simulink model "controller"  (R2016b)
settings: Solver=VariableStepAuto  StartTime=0.0  StopTime=10.0  RelTol=1e-3
values from neighbouring files (symbols this model uses):
  MAX_TORQUE_OUTPUT = 500    [Control_Init.m]
  PID_D = 0.01    [Control_Init.m]
  PID_I = 0.0    (= 0)    [Control_Init.m]
  PID_P = 0.2    [Control_Init.m]
undefined symbols (not defined in the file or in its folder): PID_FN
libraries: simulink x2
settings Model: Creator=root  LastModifiedBy=root
settings DataIOCC: SignalLogging=off
settings HardwareCC: ProdBitPerLong=64  ProdHWDeviceType=Intel->x86-64 (Linux 64)
settings RTWCC: GenCodeOnly=on  PackageGeneratedCodeAndArtifacts=on  PackageName=library

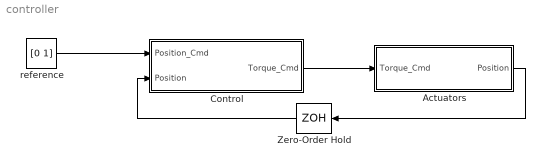
== system controller ==
  Actuators : Subsystem
  Control : Subsystem
  Zero-Order Hold : ZeroOrderHold  SampleTime=0.001
  reference : Constant  Value=[0 1]
  wires:
  Control/1(Torque_Cmd) -> Actuators/1(Torque_Cmd)
  Actuators/1(Position) -> Zero-Order Hold/1
  reference/1 -> Control/1(Position_Cmd)
  Zero-Order Hold/1 -> Control/2(Position)

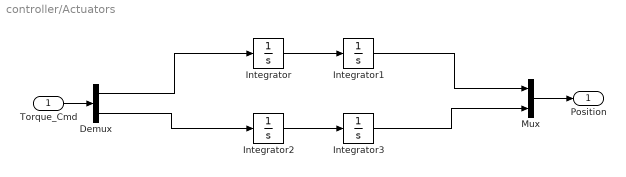
== system controller/Actuators ==
  Torque_Cmd : Inport
  Demux : Demux  Outputs=2
  Integrator : Integrator  ContinuousStateAttributes='velocity_1'
  Integrator1 : Integrator  ContinuousStateAttributes='position_1'
  Integrator2 : Integrator  ContinuousStateAttributes='velocity_2'
  Integrator3 : Integrator  ContinuousStateAttributes='position_2'
  Mux : Mux  Inputs=2
  Position : Outport
  wires:
  Integrator/1 -> Integrator1/1
  Integrator2/1 -> Integrator3/1
  Demux/1 -> Integrator/1
  Mux/1 -> Position/1
  Integrator1/1 -> Mux/1
  Integrator3/1 -> Mux/2
  Demux/2 -> Integrator2/1
  Torque_Cmd/1 -> Demux/1

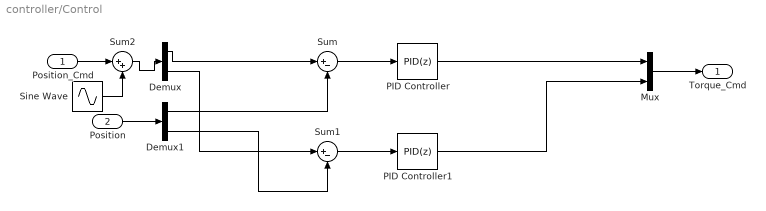
== system controller/Control ==
  Position_Cmd : Inport  PortDimensions=n_actuators
  Position : Inport  Port=2  PortDimensions=n_actuators
  Demux : Demux  Outputs=n_actuators
  Demux1 : Demux  Outputs=n_actuators
  Mux : Mux  Inputs=n_actuators
  PID Controller : simulink/Continuous/PID Controller  Controller=PID  TimeDomain=Discrete-time  SampleTime=-1  IntegratorMethod=Forward Euler  FilterMethod=Forward Euler  Form=Parallel  UseFilter=on  ControllerParametersSource=internal  P=PID_P  I=PID_I  D=PID_D  N=PID_FN  InitialConditionSource=internal  InitialConditionForIntegrator=0  InitialConditionForFilter=0  ExternalReset=none  LimitOutput=on  UpperSaturationLimit=MAX_TORQUE_OUTPUT  LowerSaturationLimit=-MAX_TORQUE_OUTPUT  LinearizeAsGain=on  AntiWindupMode=clamping  Kb=1  TrackingMode=off  Kt=1  PParamMin=[]  PParamMax=[]  IParamMin=[]  IParamMax=[]  DParamMin=[]  DParamMax=[]  NParamMin=[]  NParamMax=[]  KbParamMin=[]  KbParamMax=[]  KtParamMin=[]  KtParamMax=[]  POutMin=[]  POutMax=[]  IOutMin=[]  IOutMax=[]  DOutMin=[]  DOutMax=[]  NOutMin=[]  NOutMax=[]  KbOutMin=[]  KbOutMax=[]  KtOutMin=[]  KtOutMax=[]  IntegratorOutMin=[]  IntegratorOutMax=[]  FilterOutMin=[]  FilterOutMax=[]  SumOutMin=[]  SumOutMax=[]  SumI1OutMin=[]  SumI1OutMax=[]  SumI2OutMin=[]  SumI2OutMax=[]  SumI3OutMin=[]  SumI3OutMax=[]  SumDOutMin=[]  SumDOutMax=[]  SaturationOutMin=[]  SaturationOutMax=[]  IntegratorContinuousStateAttributes=''  IntegratorStateMustResolveToSignalObject=off  IntegratorRTWStateStorageClass=Auto  FilterContinuousStateAttributes=''  FilterStateMustResolveToSignalObject=off  FilterRTWStateStorageClass=Auto  DifferentiatorICPrevScaledInput=0  DifferentiatorOutMin=[]  DifferentiatorOutMax=[]
  PID Controller1 : simulink/Continuous/PID Controller  Controller=PID  TimeDomain=Discrete-time  SampleTime=-1  IntegratorMethod=Forward Euler  FilterMethod=Forward Euler  Form=Parallel  UseFilter=on  ControllerParametersSource=internal  P=PID_P  I=PID_I  D=PID_D  N=PID_FN  InitialConditionSource=internal  InitialConditionForIntegrator=0  InitialConditionForFilter=0  ExternalReset=none  LimitOutput=on  UpperSaturationLimit=MAX_TORQUE_OUTPUT  LowerSaturationLimit=-MAX_TORQUE_OUTPUT  LinearizeAsGain=on  AntiWindupMode=clamping  Kb=1  TrackingMode=off  Kt=1  PParamMin=[]  PParamMax=[]  IParamMin=[]  IParamMax=[]  DParamMin=[]  DParamMax=[]  NParamMin=[]  NParamMax=[]  KbParamMin=[]  KbParamMax=[]  KtParamMin=[]  KtParamMax=[]  POutMin=[]  POutMax=[]  IOutMin=[]  IOutMax=[]  DOutMin=[]  DOutMax=[]  NOutMin=[]  NOutMax=[]  KbOutMin=[]  KbOutMax=[]  KtOutMin=[]  KtOutMax=[]  IntegratorOutMin=[]  IntegratorOutMax=[]  FilterOutMin=[]  FilterOutMax=[]  SumOutMin=[]  SumOutMax=[]  SumI1OutMin=[]  SumI1OutMax=[]  SumI2OutMin=[]  SumI2OutMax=[]  SumI3OutMin=[]  SumI3OutMax=[]  SumDOutMin=[]  SumDOutMax=[]  SaturationOutMin=[]  SaturationOutMax=[]  IntegratorContinuousStateAttributes=''  IntegratorStateMustResolveToSignalObject=off  IntegratorRTWStateStorageClass=Auto  FilterContinuousStateAttributes=''  FilterStateMustResolveToSignalObject=off  FilterRTWStateStorageClass=Auto  DifferentiatorICPrevScaledInput=0  DifferentiatorOutMin=[]  DifferentiatorOutMax=[]
  Sine Wave : Sin  Amplitude=[10000 10000]  SampleTime=0
  Sum : Sum  Inputs=|+-
  Sum1 : Sum  Inputs=|+-
  Sum2 : Sum  Inputs=|++
  Torque_Cmd : Outport  PortDimensions=n_actuators
  wires:
  Demux1/1 -> Sum/2
  Sum/1 -> PID Controller/1
  Demux1/2 -> Sum1/2
  Sum1/1 -> PID Controller1/1
  Demux/1 -> Sum/1
  Demux/2 -> Sum1/1
  Position/1 -> Demux1/1
  PID Controller/1 -> Mux/1
  PID Controller1/1 -> Mux/2
  Mux/1 -> Torque_Cmd/1
  Sine Wave/1 -> Sum2/2
  Position_Cmd/1 -> Sum2/1
  Sum2/1 -> Demux/1
